simulink model "Square_Timing_Recovery"  (R2022a)
settings: Solver=FixedStepDiscrete  StartTime=0  StopTime=inf  RelTol=1e-3  EnableMultiTasking=on
undefined symbols (not defined in the file): gcbh, magnitude, rcfiltgaincompat
libraries: commfilt2 x2, commchan3 x1, dspsigops x1, simulink x1, commdigbbndpm3 x1, commrandsrc2 x1, dspxfrm3 x1, dspobslib x1
settings Model: Creator=schwall  LastModifiedBy=charlotte
settings SolverCC: AlgebraicLoopSolver=TrustRegion
settings DataIOCC: LimitDataPoints=on  SaveFormat=Array  SignalLoggingSaveFormat=ModelDataLogs  SaveOutput=off  SignalLogging=off  SaveTime=off  ReturnWorkspaceOutputs=off
settings OptimizationCC: ExpressionDepthLimit=2147483647  LifeSpan=inf
settings DebuggingCC: UnderspecifiedInitializationDetection=Classic  MergeDetectMultiDrivingBlocksExec=none  SolverPrmCheckMsg=warning  FcnCallInpInsideContextMsg=warning  UnconnectedInputMsg=warning  UnconnectedOutputMsg=warning  UnconnectedLineMsg=warning  AllowSymbolicDim=off  StateNameClashWarn=warning  SFUnexpectedBacktrackingDiag=warning  SFNoUnconditionalDefaultTransitionDiag=warning  SFExecutionAtInitializationDiag=none  SFMachineParentedDataDiag=warning  ArithmeticOperatorsInVariantConditions=warning
settings HardwareCC: ProdBitPerPointer=32  ProdBitPerSizeT=32  ProdBitPerPtrDiffT=32  ProdLargestAtomicFloat=None  ProdIntDivRoundTo=Undefined  ProdEndianess=Unspecified  ProdWordSize=32  ProdHWDeviceType=32-bit Generic
settings ModelReferenceCC: PropagateSignalLabelsOutOfModel=off
settings SFSimCC: SimUseLocalCustomCode=off  SimParseCustomCode=off  CustomCodeUndefinedFunction=UseInterfaceOnly
settings RTWCC: RTWUseLocalCustomCode=off
settings CodeAppCC: StateflowObjectComments=on
settings GRTTargetCC: TargetLangStandard=C89/C90 (ANSI)  CombineOutputUpdateFcns=off  GRTInterface=on
settings ConfigComp: CovMetricSettings=dw  CovSaveCumulativeToWorkspaceVar=on  CovSaveSingleToWorkspaceVar=on  CovExternalEMLEnable=off  CovSFcnEnable=off

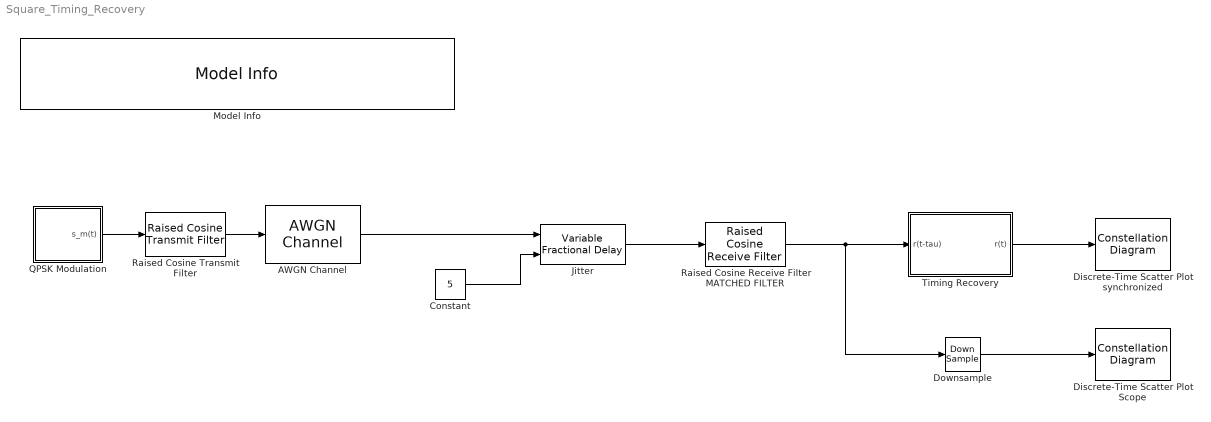
== system Square_Timing_Recovery ==
  AWGN Channel : commchan3/AWGN Channel  InputProcessing=Columns as channels (frame based)  seed=67  noiseMode="Signal to noise ratio  (Es/No)"  EbNodB=10  EsNodB=20  SNRdB=100  bitsPerSym=1  Ps=1/8  Tsym=1/1000  variance=1
  Constant : Constant  Value=5
  Discrete-Time Scatter Plot Scope : ConstellationDiagram  Tag=ScatterPlot  WindowPosition=[89.000000,465.000000,428.000000,416.000000,]  ScopeFrameLocation=window  SymbolsToDisplaySource=Property  SymbolsToDisplay=40  Title=Scatter Plot  XLimits=[-3.3 3.315]  YLimits=[-3.3 3.315]  ShowReferenceConstellation=off  ColorFading=on  DefaultConfigurationName=comm.scopes.ConstellationDiagramBlockCfg
  Discrete-Time Scatter Plot synchronized : ConstellationDiagram  Tag=ScatterPlot  WindowPosition=[94.000000,12.000000,428.000000,416.000000,]  ScopeFrameLocation=window  SymbolsToDisplaySource=Property  SymbolsToDisplay=40  Title=Scatter Plot  XLimits=[-3.3 3.315]  YLimits=[-3.3 3.315]  ShowReferenceConstellation=off  ColorFading=on  DefaultConfigurationName=comm.scopes.ConstellationDiagramBlockCfg
  Downsample : DownSample  N=8  InputProcessing=Inherited (this choice will be removed - see release notes)  RateOptions=Allow multirate processing
  Jitter : dspsigops/Variable Fractional Delay  mode=OBSOLETE  modeActive=Linear  L=4  FarrowL=4  R=10  alpha=1  dmax=100  InputProcessing=Columns as channels (frame based)  ic=0  noDFT=off  fallbackFIR=Clip to the minimum value necessary for centered kernel  fallbackFarrow=Clip to the minimum value necessary for centered kernel  roundingMode=Zero  overflowMode=off
      settings: SourceProductBaseCode=DS
  Model Info : simulink/Model-Wide Utilities/Model Info  Frame=on  DisplayStringWithTags=|  HorizontalTextAlignment=Left  LeftAlignmentValue=0.02
      | Demo Square Timing Recovery
      | Vorlesung Nachrichtentechnik II
      | Institut fuer Nachrichtentechnik (CEL)
  QPSK Modulation : Subsystem
  Raised Cosine Receive Filter MATCHED FILTER : commfilt2/Raised Cosine Receive Filter  filtType=Square root  R=1  filtSpan=2*(4)  N=8  downFactor=1  downOffset=0  filterGain=(1)*rcfiltgaincompat(gcbh)  InputProcessing=Columns as channels (frame based)  RateOptions=Enforce single-rate processing  framing=Mute  checkCoeff=off  variableName=rcRxFilt  currentFiltSpan=2*(4)  D=4  inputOffset=0  sampMode=Mute  saveAsFlag=0  rateMode=Downsampling  checkGain=User-specified  launchFVT=off  roundingMode=Floor  overflowMode=off  coeffDataTypeStr=Inherit: Same word length as input  coeffMin=[]  coeffMax=[]  coeffLastDataTypeStr=Inherit: Same word length as input  accumDataTypeStr=Inherit: Same as product output  accumLastDataTypeStr=Inherit: Same as product output  outputDataTypeStr=Inherit: Same as accumulator  outputMin=[]  outputMax=[]  outputLastDataTypeStr=Inherit: Same as accumulator
  Raised Cosine Transmit Filter : commfilt2/Raised Cosine Transmit Filter  filtType=Square root  R=1  filtSpan=2*(4)  N=8  filterGain=(1)*rcfiltgaincompat(gcbh)  InputProcessing=Columns as channels (frame based)  RateOptions=Enforce single-rate processing  framing=Mute  checkCoeff=off  variableName=rcTxFilt  checkGain=User-specified  sampMode=Mute  saveAsFlag=0  currentFiltSpan=2*(4)  D=4  launchFVT=off  roundingMode=Floor  overflowMode=off  coeffDataTypeStr=Inherit: Same word length as input  coeffMin=[]  coeffMax=[]  coeffLastDataTypeStr=Inherit: Same word length as input  outputDataTypeStr=Inherit: Same as accumulator  outputMin=[]  outputMax=[]  outputLastDataTypeStr=Inherit: Same as accumulator
  Timing Recovery : Subsystem
  wires:
  QPSK Modulation/1(s_m(t)) -> Raised Cosine Transmit Filter/1
  Downsample/1 -> Discrete-Time Scatter Plot Scope/1
  Raised Cosine Transmit Filter/1 -> AWGN Channel/1
  Raised Cosine Receive Filter MATCHED FILTER/1 -> Downsample/1, Timing Recovery/1(r(t-tau))
  Timing Recovery/1(r(t)) -> Discrete-Time Scatter Plot synchronized/1
  Constant/1 -> Jitter/2
  AWGN Channel/1 -> Jitter/1
  Jitter/1 -> Raised Cosine Receive Filter MATCHED FILTER/1

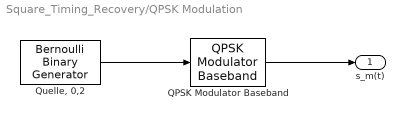
== system Square_Timing_Recovery/QPSK Modulation ==
  QPSK Modulator Baseband : commdigbbndpm3/QPSK Modulator Baseband  InType=Bit  Enc=Binary  Ph=pi/4  outDtype=double  outWordLen=16  outUDDataType=sfix(16)  outFracLenMode=Best precision  outFracLen=15  outDataTypeStr=double  outLastDataTypeStr=double
  "Quelle, 0,2" : commrandsrc2/Bernoulli Binary Generator  P=0.5  seed=61  Ts=1/1000/2  frameBased=on  sampPerFrame=128  orient=off  outDataType=double
      settings: SourceProductBaseCode=CM
  s_m(t) : Outport
  wires:
  "Quelle, 0,2"/1 -> QPSK Modulator Baseband/1
  QPSK Modulator Baseband/1 -> s_m(t)/1

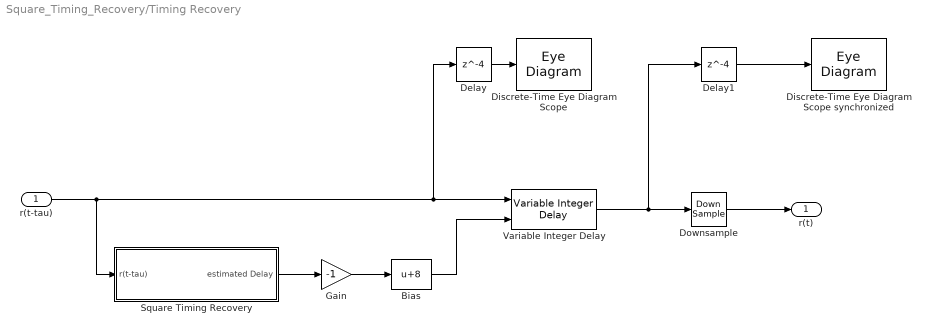
== system Square_Timing_Recovery/Timing Recovery ==
  r(t-tau) : Inport
  Bias : Bias  Bias=8  SaturateOnIntegerOverflow=off
  Delay : Delay  DelayLength=4  InitialCondition=0  InputProcessing=Columns as channels (frame based)
  Delay1 : Delay  DelayLength=4  InitialCondition=0  InputProcessing=Columns as channels (frame based)
  Discrete-Time Eye Diagram Scope : EyeDiagram  Tag=EyeDiagram
  Discrete-Time Eye Diagram Scope synchronized : EyeDiagram  Tag=EyeDiagram
  Downsample : DownSample  N=8  InputProcessing=Inherited (this choice will be removed - see release notes)  RateOptions=Allow multirate processing
  Gain : Gain  Gain=-1
  Square Timing Recovery : Subsystem
  Variable Integer Delay : dspobslib/Variable Integer Delay  dmax=100  InputProcessing=Columns as channels (frame based)  ic=0  noDFT=off
      settings: SourceProductBaseCode=DS
  r(t) : Outport
  wires:
  r(t-tau)/1 -> Square Timing Recovery/1(r(t-tau)), Delay/1, Variable Integer Delay/1
  Square Timing Recovery/1(estimated Delay) -> Gain/1
  Gain/1 -> Bias/1
  Bias/1 -> Variable Integer Delay/2
  Variable Integer Delay/1 -> Delay1/1, Downsample/1
  Downsample/1 -> r(t)/1
  Delay1/1 -> Discrete-Time Eye Diagram Scope synchronized/1
  Delay/1 -> Discrete-Time Eye Diagram Scope/1

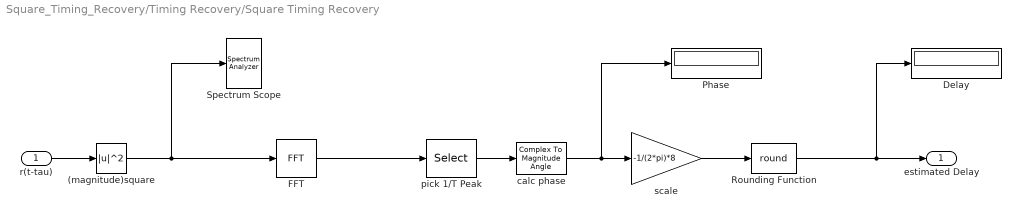
== system Square_Timing_Recovery/Timing Recovery/Square Timing Recovery ==
  r(t-tau) : Inport
  (magnitude)square : Math  Operator=magnitude^2  SignedPower=on
  Delay : Display
  FFT : dspxfrm3/FFT  FFTImplementation=Auto  CompMethod=Table lookup  TableOpt=NEW  TableOptActive=Speed  BitRevOrder=off  Normalize=off  InheritFFTLength=on  FFTLength=64  WrapInput=on  roundingMode=Floor  overflowMode=off  firstCoeffDataTypeStr=Inherit: Same word length as input  firstCoeffLastDataTypeStr=Inherit: Same word length as input  outputMin=[]  outputMax=[]
  Phase : Display
  Rounding Function : Rounding  Operator=round
  Spectrum Scope : SpectrumAnalyzer
  calc phase : ComplexToMagnitudeAngle  Output=Angle
  pick 1/T Peak : Selector  InputPortWidth=512  IndexOptions=Index vector (dialog)  Indices=[65]  OutputSizes=1
  scale : Gain  Gain=-1/(2*pi)*8
  estimated Delay : Outport
  wires:
  (magnitude)square/1 -> FFT/1, Spectrum Scope/1
  FFT/1 -> pick 1/T Peak/1
  pick 1/T Peak/1 -> calc phase/1
  calc phase/1 -> scale/1, Phase/1
  scale/1 -> Rounding Function/1
  r(t-tau)/1 -> (magnitude)square/1
  Rounding Function/1 -> estimated Delay/1, Delay/1
